simulink model "schemat_koncowy_irp"  (R2015a)
settings: Solver=ode1  StartTime=0.0  StopTime=Inf  FixedStep=0.001  RelTol=1e-3
PostLoadFcn:
  | , if any(exist('dsrtsu_mdlpostloadfcn', 'file') == [2, 3, 6]), try dsrtsu_mdlpostloadfcn('Execute', bdroot); catch fprintf('Error in PostLoadFcn (dsrtsu_mdlpostloadfcn) for model "%s":\n %s\n', bdroot, lasterr); end, end,
libraries: rtilibm x3
(part 1 of 2)
settings Model: DSRTSU_INTERNAL_RTI_VER=460  DSRTSU_INTERNAL_RTI_TYPE=rti1005  DSRTSU_INTERNAL_RTIFPGA=50  CovHtmlReporting=off  Creator=k21p930a  LastModifiedBy=k21p930a
settings OptimizationCC: BlockReduction=off  OptimizeBlockIOStorage=off  BufferReuse=off  GlobalBufferReuse=off  ExpressionFolding=off  LocalBlockOutputs=off
settings HardwareCC: ProdIntDivRoundTo=Zero  ProdEndianess=BigEndian  ProdHWDeviceType=Generic->Custom  TargetIntDivRoundTo=Zero  TargetEndianess=BigEndian  TargetHWDeviceType=Generic->Custom
settings RTWCC: SystemTargetFile=rti1005.tlc  MakeCommand=make_rti  TemplateMakefile=rti1005.tmf  Description=dSPACE DS1005 Hardware Platform
settings STFCustomTargetCC: GenerateSampleERTMain=off  ParMdlRefBuildCompliant=on  GeneratePreprocessorConditionals=Disable all  ERTCustomFileBanners=off  SupportNonInlinedSFcns=on  SupportVariableSizeSignals=off  MATLABClassNameForMDSCustomization=Simulink.SoftwareTarget.GRTCustomization  GRTInterface=on  SystemTargetFile=rti1005.tlc
settings GRTTargetCC: CompOptLevelCompliant=off  ConcurrentExecutionCompliant=off  CombineOutputUpdateFcns=off  MatFileLogging=off  CPPClassGenCompliant=off  GRTInterface=on  ExtModeMexFile=noextcomm

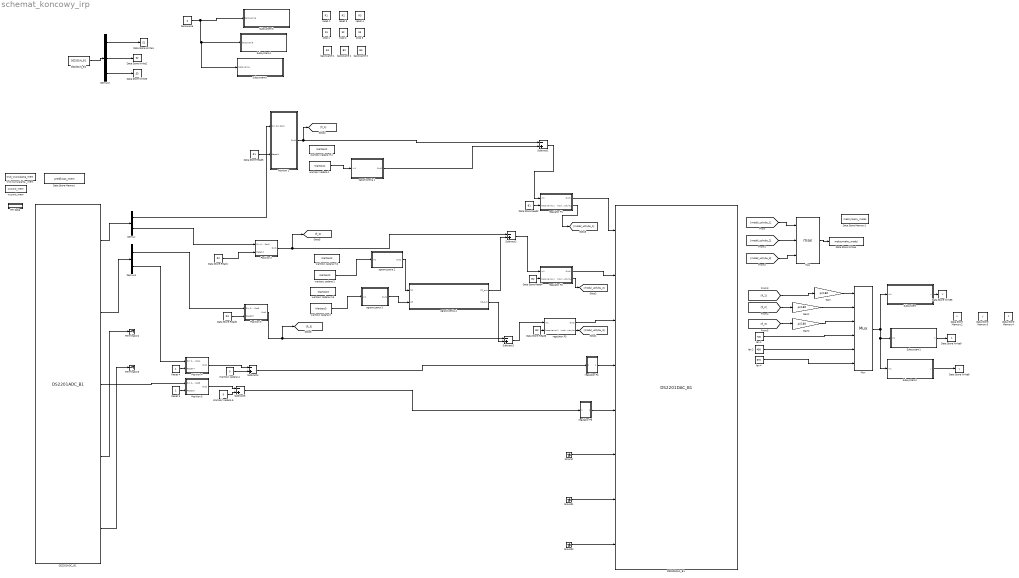
== system schemat_koncowy_irp ==
  DS2201ADC_B1 : rtilibm/DS2201/DS2201ADC_B1  BoardNo=1  channelNo1=[1 2 3 4]  channelNo2=[5 6 7 8]  channelNo3=[9 10]  channelNo4=-1  channelNo5=-1  DialogFcn=gui2201adc  UnitName={'DS2201ADC_B'}  UnitValues={ 1 }  DSProperties=struct('RTI',struct('Version',uint32(1),'BlockType',struct('isSLSource',uint8(1),'isSLSink',uint8(0),'isHWSource',uint8(1),'isHWSink',uint8(0),'isSetup',uint8(0),'isInline',uint8(1),'isNonInline',uint8(0),'isInterrupt',uint8(0),'isChannelwise',uint8(0)),'IOBoardType','DS2201','UnitType','ADC','Identifier','ADCMUX','DialogType','ML','BlockSet','NONE','SlaveProcessor','NONE'))
  DS2201DAC_B1 : rtilibm/DS2201/DS2201DAC_B1  BoardNo=1  IOErrorMode=[0 0]  InitValue=[0 0 0 0 0 0 0 0]  TermMode=[0 0 0 0 0 0 0 0]  TermValue=[0 0 0 0 0 0 0 0]  DialogFcn=gui2201dac  UnitName={'DS2201DAC_B'}  UnitValues={ 1 }  DSProperties=struct('RTI',struct('Version',uint32(1),'BlockType',struct('isSLSource',uint8(0),'isSLSink',uint8(1),'isHWSource',uint8(0),'isHWSink',uint8(1),'isSetup',uint8(0),'isInline',uint8(1),'isNonInline',uint8(0),'isInterrupt',uint8(0),'isChannelwise',uint8(0)),'IOBoardType','DS2201','UnitType','DAC','Identifier','DAC','DialogType','ML','BlockSet','NONE','SlaveProcessor','NONE'))
  DS2201IN_B1 : rtilibm/DS2201/DS2201IN_B1  BoardNo=1  ChannelNos=[1 2 3]  DialogFcn=gui2201in  UnitName={ 'DS2201IN_B' }  UnitValues={ 1 }  DSProperties=struct('RTI',struct('Version',uint32(1),'BlockType',struct('isSLSource',uint8(1),'isSLSink',uint8(0),'isHWSource',uint8(1),'isHWSink',uint8(0),'isSetup',uint8(0),'isInline',uint8(1),'isNonInline',uint8(0),'isInterrupt',uint8(0),'isChannelwise',uint8(0)),'IOBoardType','DS2201','UnitType','BIT','Identifier','BITIN','DialogType','ML','BlockSet','NONE','SlaveProcessor','NONE'))
  Data Store Memory : DataStoreMemory  DataStoreName=predkosc_mem  ReadBeforeWriteMsg=warning  WriteAfterWriteMsg=warning  WriteAfterReadMsg=warning  InitialValue=0.3
  Data Store Memory1 : DataStoreMemory  DataStoreName=maksymalny_modul  ReadBeforeWriteMsg=warning  WriteAfterWriteMsg=warning  WriteAfterReadMsg=warning
  Data Store Memory2 : DataStoreMemory  DataStoreName=x  ReadBeforeWriteMsg=warning  WriteAfterWriteMsg=warning  WriteAfterReadMsg=warning
  Data Store Memory3 : DataStoreMemory  DataStoreName=y  ReadBeforeWriteMsg=warning  WriteAfterWriteMsg=warning  WriteAfterReadMsg=warning
  Data Store Memory4 : DataStoreMemory  DataStoreName=z  ReadBeforeWriteMsg=warning  WriteAfterWriteMsg=warning  WriteAfterReadMsg=warning
  Data Store Read1 : DataStoreRead  DataStoreName=R2
  Data Store Read2 : DataStoreRead  DataStoreName=B1
  Data Store Read3 : DataStoreRead  DataStoreName=R3
  Data Store Read4 : DataStoreRead  DataStoreName=B2
  Data Store Read5 : DataStoreRead  DataStoreName=R1
  Data Store Read6 : DataStoreRead  DataStoreName=B3
  Data Store Write1 : DataStoreWrite  DataStoreName=S1
  Data Store Write2 : DataStoreWrite  DataStoreName=S2
  Data Store Write3 : DataStoreWrite  DataStoreName=S3
  Data Store Write4 : DataStoreWrite  DataStoreName=maksymalny_modul
  Data Store Write5 : DataStoreWrite  DataStoreName=x
  Data Store Write8 : DataStoreWrite  DataStoreName=y
  Data Store Write9 : DataStoreWrite  DataStoreName=z
  Demux : Demux  Outputs=2
  Demux1 : Demux  Outputs=2
  Demux2 : Demux  Outputs=3
  Gain : Gain  Gain=pi/180
  Gain1 : Gain  Gain=pi/180
  Gain2 : Gain  Gain=pi/180
  Ground : Ground
  Ground1 : Ground
  Ground2 : Ground
  Max : MinMax  Function=max  Inputs=3
  Mux : Mux  Inputs=6
  Position 1 : Subsystem
  Position 2 : Subsystem
  Position 3 : Subsystem
  Position 4 : Subsystem
  Position 5 : Subsystem
  RTI Data : Subsystem  Tag=struct('RTIDataServer',struct('RTIDataServerVs','2','RTIModelDescription','struct(''main'',''schemat_koncowy_irp'',''sub'',''schemat_koncowy_irp'',''isMp'',0)'))  LoadFcn="if exist('rtidc'), try,  rtidc('DataHostBlockClbLoad', gcbh); catch, disp(['Warning: ''LoadFcn'' for RTI Data block failed: ' lasterr]); end, end,"  mask(RTI_DATA_HOST){}
      mask help:
      | RTI Data Block.
      | This block is used by RTI to store internal model-dependent data.
      | Please keep this block on the root level of the model. Deleting this block will result in data loss.
      |
      | NEVER DELETE OR COPY THIS BLOCK!
      settings: CopyFcn="if exist('rtidc'), try,  rtidc('DataHostBlockClbCopy', gcbh); catch, disp(['Warning: ''CopyFcn'' for RTI Data block failed: ' lasterr]); end, end,"  DeleteFcn="if exist('rtidc'), try,  rtidc('DataHostBlockClbDelete', gcbh); catch, disp(['Warning: ''DeleteFcn'' for RTI Data block failed: ' lasterr]); end, end,"  ModelCloseFcn="if exist('rtidc'), try,  rtidc('DataHostBlockClbModelClose', gcbh); catch, disp(['Warning: ''ModelCloseFcn'' for RTI Data block failed: ' lasterr]); end, end,"  PreSaveFcn="if exist('rtidc'), try,  rtidc('DataHostBlockClbPreSave', gcbh); catch, disp(['Warning: ''PreSaveFcn'' for RTI Data block failed: ' lasterr]); end, end,"  PostSaveFcn="if exist('rtidc'), try,  rtidc('DataHostBlockClbPostSave', gcbh); catch, disp(['Warning: ''PostSaveFcn'' for RTI Data block failed: ' lasterr]); end, end,"  NameChangeFcn="if exist('rtidc'), try,  rtidc('DataHostBlockClbNameChange', gcbh); catch, disp(['Warning: ''NameChangeFcn'' for RTI Data block failed: ' lasterr]); end, end,"
      mask Help:
      | RTI Data Block.
      | This block is used by RTI to store internal model-dependent data.
      | Please keep this block on the root level of the model. Deleting this block will result in data loss.
      | 
      | NEVER DELETE OR COPY THIS BLOCK!
      mask Display:
      | text(0.5, 0.5, 'RTI Data', 'HorizontalAlignment', 'center');
      | plot([1 0]);
  Reset 4 : Constant
  Reset 5 : Constant
  Subsystem : Subsystem
  Subsystem1 : Subsystem
  Subsystem2 : Subsystem
  Subsystem3 : Subsystem
  Subsystem4 : Subsystem
  Subsystem5 : Subsystem
  Subtract{1..5} (5 alike) : Sum  Inputs=-+
  Terminator2 : Terminator
  Terminator3 : Terminator
  Wartość zadana 4 : Constant  Value=0
  Wartość zadana 5 : Constant  Value=0
  "bazowanie " : Constant  Value=0
  bazowanie 1 : DataStoreMemory  DataStoreName=B1  ReadBeforeWriteMsg=warning  WriteAfterWriteMsg=warning  WriteAfterReadMsg=warning
  bazowanie 2 : DataStoreMemory  DataStoreName=B2  ReadBeforeWriteMsg=warning  WriteAfterWriteMsg=warning  WriteAfterReadMsg=warning
  bazowanie 3 : DataStoreMemory  DataStoreName=B3  ReadBeforeWriteMsg=warning  WriteAfterWriteMsg=warning  WriteAfterReadMsg=warning
  len 1 : Constant  Value=700
  len 2 : Constant  Value=450
  len 4 : Constant  Value=670
  ograniczenia 1 : Subsystem
  ograniczenia 2 : Subsystem
  ograniczenia 3 : Subsystem
  ograniczenia 4 : Subsystem
  regulator P1 : Subsystem
  regulator P2 : Subsystem
  regulator P3 : Subsystem
  regulator P4 : Subsystem
  regulator P5 : Subsystem
  reset 1 : DataStoreMemory  DataStoreName=R1  ReadBeforeWriteMsg=warning  WriteAfterWriteMsg=warning  WriteAfterReadMsg=warning  OutDataTypeStr=double
  reset 3 : DataStoreMemory  DataStoreName=R2  ReadBeforeWriteMsg=warning  WriteAfterWriteMsg=warning  WriteAfterReadMsg=warning  OutDataTypeStr=double
  reset 4 : DataStoreMemory  DataStoreName=R3  ReadBeforeWriteMsg=warning  WriteAfterWriteMsg=warning  WriteAfterReadMsg=warning  OutDataTypeStr=double
  stop 1 : DataStoreMemory  DataStoreName=S1  ReadBeforeWriteMsg=warning  WriteAfterWriteMsg=warning  WriteAfterReadMsg=warning
  stop 2 : DataStoreMemory  DataStoreName=S2  ReadBeforeWriteMsg=warning  WriteAfterWriteMsg=warning  WriteAfterReadMsg=warning
  stop 3 : DataStoreMemory  DataStoreName=S3  ReadBeforeWriteMsg=warning  WriteAfterWriteMsg=warning  WriteAfterReadMsg=warning
  "tryb wyzwalania _mem " : DataStoreMemory  DataStoreName=tryb_wyzwalania_mem  ReadBeforeWriteMsg=warning  WriteAfterWriteMsg=warning  WriteAfterReadMsg=warning
  wartosc zadana 1 : DataStoreRead  DataStoreName=Wartosc1
  wartosc zadana 2 : DataStoreRead  DataStoreName=Wartosc2
  wartosc zadana 3 : DataStoreRead  DataStoreName=Wartosc3
  wartosc zadana m1 : DataStoreMemory  DataStoreName=Wartosc1  ReadBeforeWriteMsg=warning  WriteAfterWriteMsg=warning  WriteAfterReadMsg=warning
  wartosc zadana m2 : DataStoreMemory  DataStoreName=Wartosc2  ReadBeforeWriteMsg=warning  WriteAfterWriteMsg=warning  WriteAfterReadMsg=warning
  wartosc zadana m3 : DataStoreMemory  DataStoreName=Wartosc3  ReadBeforeWriteMsg=warning  WriteAfterWriteMsg=warning  WriteAfterReadMsg=warning
  wyzwol_mem : DataStoreMemory  DataStoreName=wyzwol_mem  ReadBeforeWriteMsg=warning  WriteAfterWriteMsg=warning  WriteAfterReadMsg=warning
  wires:
  Demux1/2 -> Position 4/1(Sin && Cos4)
  DS2201ADC_B1/1 -> Demux/1
  DS2201ADC_B1/2 -> Demux1/1
  DS2201ADC_B1/5 -> Terminator3/1
  DS2201ADC_B1/4 -> Terminator2/1
  Demux/1 -> Position 1/1(Sin && Cos1)
  Demux/2 -> Position 2/1(Sin && Cos2)
  Demux1/1 -> Position 3/1(Sin && Cos3)
  DS2201ADC_B1/3 -> Position 5/1(Sin && Cos5)
  regulator P1/1(Out1) -> DS2201DAC_B1/1
  regulator P4/1(Out1) -> DS2201DAC_B1/4
  regulator P5/1(Out1) -> DS2201DAC_B1/5
  wartosc zadana 1/1 -> ograniczenia 1/1(In1)
  Position 1/1(Out1) -> [fi_1], Subtract1/1
  Position 2/1(Out1) -> [fi_2], Subtract2/1
  Position 3/1(Out1) -> [fi_3], Subtract3/1
  Position 4/1(Out1) -> Subtract4/1
  Position 5/1(Out1) -> Subtract5/1
  Subtract5/1 -> regulator P5/1(In1)
  Subtract4/1 -> regulator P4/1(In1)
  Ground/1 -> DS2201DAC_B1/6
  Ground1/1 -> DS2201DAC_B1/7
  Ground2/1 -> DS2201DAC_B1/8
  Wartość zadana 4/1 -> Subtract4/2
  Wartość zadana 5/1 -> Subtract5/2
  Reset 4/1 -> Position 4/2(Reset 4)
  Reset 5/1 -> Position 5/2(Reset 5)
  DS2201IN_B1/1 -> Demux2/1
  ograniczenia 1/1(Out1) -> Subtract1/2
  Subtract1/1 -> regulator P1/1(In1)
  ograniczenia 2/1(Out1) -> ograniczenia 4/1(Z2)
  ograniczenia 4/1(Z2_out) -> Subtract2/2
  ograniczenia 3/1(Out1) -> ograniczenia 4/2(Z3)
  ograniczenia 4/2("Z3_out ") -> Subtract3/2
  Demux2/1 -> Data Store Write1/1
  Demux2/2 -> Data Store Write2/1
  Demux2/3 -> Data Store Write3/1
  Data Store Read3/1 -> Position 3/2(Reset 3)
  Data Store Read5/1 -> Position 1/2(Reset 1)
  Data Store Read2/1 -> regulator P1/2(bazowanie 1)
  regulator P2/1(Out1) -> DS2201DAC_B1/2
  Subtract2/1 -> regulator P2/1(In1)
  regulator P3/1(Out1) -> DS2201DAC_B1/3
  Subtract3/1 -> regulator P3/1(In1)
  regulator P3/2(modul uchybu) -> [modul_uchybu_3]
  regulator P2/2(modul uchybu) -> [modul_uchybu_2]
  regulator P1/2(modul uchybu) -> [modul_uchybu_1]
  [modul_uchybu_1] -> Max/1
  [modul_uchybu_2] -> Max/2
  [modul_uchybu_3] -> Max/3
  Max/1 -> Data Store Write4/1
  [fi_1] -> Gain/1
  [fi_2] -> Gain1/1
  [fi_3] -> Gain2/1
  len 1/1 -> Mux/4
  len 2/1 -> Mux/5
  len 4/1 -> Mux/6
  Mux/1 -> Subsystem/1(In1), Subsystem2/1(In1), Subsystem1/1(In1)
  Subsystem/1(x) -> Data Store Write5/1
  Subsystem2/1(y) -> Data Store Write8/1
  Gain1/1 -> Mux/2
  Gain2/1 -> Mux/3
  Gain/1 -> Mux/1
  "bazowanie "/1 -> Subsystem5/1(bazowanie), Subsystem4/1(bazowanie), Subsystem3/1(bazowanie)
  Data Store Read1/1 -> Position 2/2(Reset 2)
  Data Store Read4/1 -> regulator P2/2(bazowanie 1)
  Data Store Read6/1 -> regulator P3/2(bazowanie 1)
  wartosc zadana 3/1 -> ograniczenia 3/1(In1)
  wartosc zadana 2/1 -> ograniczenia 2/1(In1)
  Subsystem1/1(z) -> Data Store Write9/1

== system schemat_koncowy_irp/Position 1 ==
  Sin && Cos1 : Inport
  Reset 1 : Inport  Port=2
  Filters 1 : Subsystem
  Position Calculation 1 : Subsystem
  Out1 : Outport
  wires:
  Filters 1/1(Sin) -> Position Calculation 1/1(Sin)
  Filters 1/2(Cos) -> Position Calculation 1/2(Cos)
  Sin && Cos1/1 -> Filters 1/1(Sin && Cos)
  Reset 1/1 -> Position Calculation 1/3(Reset (Impulse))
  Position Calculation 1/1(Position) -> Out1/1

== system schemat_koncowy_irp/Position 2 ==
  Sin && Cos2 : Inport
  Reset 2 : Inport  Port=2
  Filters 2 : Subsystem
  Position Calculation 2 : Subsystem
  Out1 : Outport
  wires:
  Filters 2/1(Sin) -> Position Calculation 2/1(Sin)
  Filters 2/2(Cos) -> Position Calculation 2/2(Cos)
  Sin && Cos2/1 -> Filters 2/1(Sin && Cos)
  Reset 2/1 -> Position Calculation 2/3(Reset (Impulse))
  Position Calculation 2/1(Position) -> Out1/1

== system schemat_koncowy_irp/Position 3 ==
  Sin && Cos3 : Inport
  Reset 3 : Inport  Port=2
  Filters 3 : Subsystem
  Position Calculation 3 : Subsystem
  Out1 : Outport
  wires:
  Filters 3/1(Sin) -> Position Calculation 3/1(Sin)
  Filters 3/2(Cos) -> Position Calculation 3/2(Cos)
  Sin && Cos3/1 -> Filters 3/1(Sin && Cos)
  Reset 3/1 -> Position Calculation 3/3(Reset (Impulse))
  Position Calculation 3/1(Position) -> Out1/1

== system schemat_koncowy_irp/Position 4 ==
  Sin && Cos4 : Inport
  Reset 4 : Inport  Port=2
  Filters 4 : Subsystem
  Position Calculation 4 : Subsystem
  Out1 : Outport
  wires:
  Position Calculation 4/1(Position) -> Out1/1
  Reset 4/1 -> Position Calculation 4/3(Reset (Impulse))
  Sin && Cos4/1 -> Filters 4/1(Sin && Cos)
  Filters 4/2(Cos) -> Position Calculation 4/2(Cos)
  Filters 4/1(Sin) -> Position Calculation 4/1(Sin)

== system schemat_koncowy_irp/Position 5 ==
  Sin && Cos5 : Inport
  Reset 5 : Inport  Port=2
  Filters 5 : Subsystem
  Position Calculation 5 : Subsystem
  Out1 : Outport
  wires:
  Position Calculation 5/1(Position) -> Out1/1
  Reset 5/1 -> Position Calculation 5/3(Reset (Impulse))
  Sin && Cos5/1 -> Filters 5/1(Sin && Cos)
  Filters 5/2(Cos) -> Position Calculation 5/2(Cos)
  Filters 5/1(Sin) -> Position Calculation 5/1(Sin)

== system schemat_koncowy_irp/RTI Data ==
  RTI Data Store : Subsystem  Tag="struct('private',struct('version',struct('dsVer',uint32(2),'dsVerCreation',uint32(2),'RTI',struct('ver','7.4','type','RTI1005')),'access',struct('type','Model','isPerm',1,'created',['18-Oct-2021 10:10:05'],'modified',['08-Nov-2021 10:46:14'],'location','')),'public',struct('main',struct('data',[]),'sub',struct('name',{{'schemat_koncowy_irp'}},'data',{{struct('TH',struct('thTaskInfo',struct('taskType',{'TIMER','HWINT','TMRINT','SWINT','GLINT'},'tasksNumOf',{1,0,0,0,0},'srcIds',{{'TIMERA'},{},{},{},{}},'taskNames',{{['Timer Task 1']},{},{},{},{}})),'th_tc',struct('dataType','TASK','taskGroupId','','taskGroupList',{{}},'taskSchedulingPolicy','FCFS','taskType','TIMER','blkh',-1,'srcId','TIMERA','srcSgnName',['Timer A interrupt'],'srcCpuName','','taskName',['Timer Task 1  [0.001] s'],'taskNameDisplayExt','','smplTime',0.001,'smplTimeOffs',0,'hasFixedPriority',0,'priority',1,'hasFixedOvc',0,'ovcType',1,'ovcMax',1),'tc_th',struct('dataType','TASK','taskGroupId','','taskGroupList',{{}},'taskSchedulingPolicy','FCFS','taskType','TIMER','blkh',-1,'srcId','TIMERA','srcSgnName',['Timer A interrupt'],'srcCpuName','','taskName',['Timer Task 1  [0.001] s'],'taskNameDisplayExt','','smplTime',0.001,'smplTimeOffs',0,'hasFixedPriority',0,'priority',1,'hasFixedOvc',0,'ovcType',1,'ovcMax',1))}})))"  mask(RTI_DATA_STORE){}
      mask help:
      | RTI Data Store Block. This block is used by RTI to store internal model dependent data. Deleting this block will result in data loss.
      |
      | NEVER DELETE, COPY, OR MODIFY THIS BLOCK!
      mask Help:
      | RTI Data Store Block. This block is used by RTI to store internal model dependent data. Deleting this block will result in data loss.
      | 
      | NEVER DELETE, COPY, OR MODIFY THIS BLOCK!
      mask Display: text(0.5, 0.5, ' ', 'HorizontalAlignment', 'center');

== system schemat_koncowy_irp/Subsystem ==
  In1 : Inport
  Cos : Trigonometry  Operator=cos
  Cos1 : Trigonometry  Operator=cos
  Demux : Demux  Outputs=6
  Product : Product
  Product1 : Product
  Product2 : Product
  Sin : Trigonometry
  Sum : Sum  Inputs=|+-
  Sum1 : Sum  Inputs=|++
  Terminator : Terminator
  x : Outport
  wires:
  Cos/1 -> Product/1
  Sum/1 -> Product/2
  Product/1 -> x/1
  Demux/2 -> Sin/1, Sum1/1  "fi2-l"
  Demux/3 -> Sum1/2
  Sum1/1 -> Cos1/1
  Cos1/1 -> Product1/1
  Demux/6 -> Product1/2  "c"
  Product1/1 -> Sum/1
  Sin/1 -> Product2/1
  Demux/5 -> Product2/2  "b"
  Product2/1 -> Sum/2
  In1/1 -> Demux/1
  Demux/1 -> Cos/1  "fi1-k"
  Demux/4 -> Terminator/1

== system schemat_koncowy_irp/Subsystem1 ==
  In1 : Inport
  Cos : Trigonometry  Operator=cos
  Demux : Demux  Outputs=6
  Product : Product
  Product1 : Product
  Sin : Trigonometry
  Sum : Sum  Inputs=3
  Sum1 : Sum  Inputs=|++
  Terminator : Terminator
  z : Outport
  wires:
  Sum/1 -> z/1
  Demux/2 -> Sum1/1, Cos/1  "fi2-l"
  Demux/3 -> Sum1/2
  In1/1 -> Demux/1
  Demux/4 -> Sum/1
  Cos/1 -> Product/1
  Demux/5 -> Product/2  "b"
  Product/1 -> Sum/2
  Sum1/1 -> Sin/1
  Sin/1 -> Product1/1
  Demux/6 -> Product1/2  "c"
  Product1/1 -> Sum/3
  Demux/1 -> Terminator/1  "fi1-k"

== system schemat_koncowy_irp/Subsystem2 ==
  In1 : Inport
  Cos : Trigonometry  Operator=cos
  Demux : Demux  Outputs=6
  Minus : Sum  Inputs=+-
  Product : Product
  Product1 : Product
  Product2 : Product
  Sin : Trigonometry
  Sin1 : Trigonometry
  Sum : Sum  Inputs=|++
  Terminator : Terminator
  y : Outport
  wires:
  Demux/2 -> Sin1/1, Sum/1  "fi2-l"
  Demux/3 -> Sum/2
  In1/1 -> Demux/1
  Demux/1 -> Sin/1  "fi1-k"
  Demux/4 -> Terminator/1
  Sin/1 -> Product/1
  Minus/1 -> Product/2
  Sin1/1 -> Product1/1
  Demux/5 -> Product1/2  "b"
  Product1/1 -> Minus/1
  Sum/1 -> Cos/1
  Cos/1 -> Product2/1
  Demux/6 -> Product2/2  "c"
  Product2/1 -> Minus/2
  Product/1 -> y/1

== system schemat_koncowy_irp/Subsystem3 ==
  bazowanie : Inport
  01 : Constant  Value=0
  4 : Constant  Value=0
  Data Store Read : DataStoreRead  DataStoreName=B1
  Data Store Read1 : DataStoreRead  DataStoreName=B1
  Data Store Read2 : DataStoreRead  DataStoreName=S1
  Data Store Write : DataStoreWrite  DataStoreName=B1
  Data Store Write2 : DataStoreWrite  DataStoreName=R1
  Data Store Write3 : DataStoreWrite  DataStoreName=Wartosc1
  Data Type Conversion : DataTypeConversion  OutDataTypeStr=double
  NOT1 : Logic  Operator=NOT  IconShape=distinctive  AllPortsSameDT=off  OutDataTypeStr=boolean
  Switch : Switch  Criteria=u2 > Threshold
  Switch1 : Switch  Criteria=u2 > Threshold
  Switch4 : Switch  Criteria=u2 > Threshold
  wartosc zadana 1 : DataStoreRead  DataStoreName=Wartosc1
  wires:
  Switch1/1 -> Data Store Write/1
  4/1 -> Switch4/1
  bazowanie/1 -> Switch/2, Switch/1
  Data Store Read/1 -> Switch/3
  NOT1/1 -> Data Type Conversion/1
  Switch/1 -> Switch1/3
  01/1 -> Switch1/1
  Switch4/1 -> Data Store Write3/1
  wartosc zadana 1/1 -> Switch4/3
  Data Store Read1/1 -> Switch4/2, NOT1/1
  Data Store Read2/1 -> Switch1/2
  Data Type Conversion/1 -> Data Store Write2/1

== system schemat_koncowy_irp/Subsystem4 ==
  bazowanie : Inport
  01 : Constant  Value=0
  4 : Constant  Value=0
  Data Store Read : DataStoreRead  DataStoreName=B2
  Data Store Read1 : DataStoreRead  DataStoreName=B2
  Data Store Read2 : DataStoreRead  DataStoreName=S2
  Data Store Write : DataStoreWrite  DataStoreName=B2
  Data Store Write2 : DataStoreWrite  DataStoreName=R2
  Data Store Write3 : DataStoreWrite  DataStoreName=Wartosc2
  Data Type Conversion : DataTypeConversion  OutDataTypeStr=double
  NOT1 : Logic  Operator=NOT  IconShape=distinctive  AllPortsSameDT=off  OutDataTypeStr=boolean
  Switch : Switch  Criteria=u2 > Threshold
  Switch1 : Switch  Criteria=u2 > Threshold
  Switch4 : Switch  Criteria=u2 > Threshold
  wartosc zadana 2 : DataStoreRead  DataStoreName=Wartosc2
  wires:
  Switch1/1 -> Data Store Write/1
  4/1 -> Switch4/1
  bazowanie/1 -> Switch/2, Switch/1
  Data Store Read/1 -> Switch/3
  NOT1/1 -> Data Type Conversion/1
  Switch/1 -> Switch1/3
  01/1 -> Switch1/1
  Switch4/1 -> Data Store Write3/1
  wartosc zadana 2/1 -> Switch4/3
  Data Store Read1/1 -> Switch4/2, NOT1/1
  Data Store Read2/1 -> Switch1/2
  Data Type Conversion/1 -> Data Store Write2/1

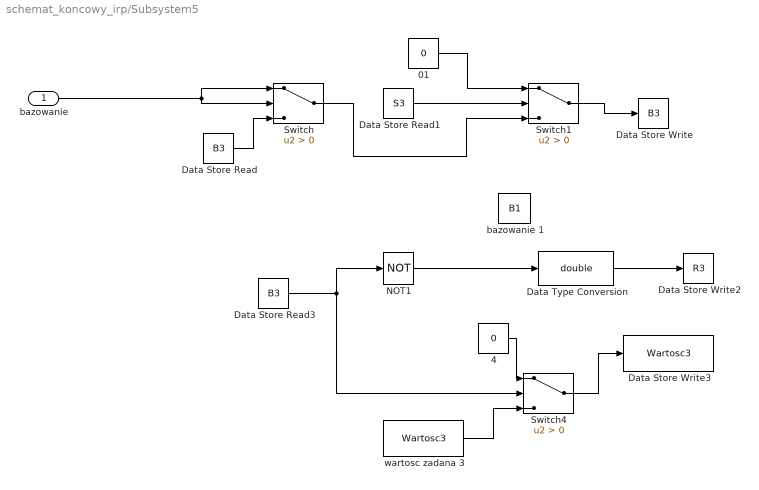
== system schemat_koncowy_irp/Subsystem5 ==
  bazowanie : Inport
  01 : Constant  Value=0
  4 : Constant  Value=0
  Data Store Read : DataStoreRead  DataStoreName=B3
  Data Store Read1 : DataStoreRead  DataStoreName=S3
  Data Store Read3 : DataStoreRead  DataStoreName=B3
  Data Store Write : DataStoreWrite  DataStoreName=B3
  Data Store Write2 : DataStoreWrite  DataStoreName=R3
  Data Store Write3 : DataStoreWrite  DataStoreName=Wartosc3
  Data Type Conversion : DataTypeConversion  OutDataTypeStr=double
  NOT1 : Logic  Operator=NOT  IconShape=distinctive  AllPortsSameDT=off  OutDataTypeStr=boolean
  Switch : Switch  Criteria=u2 > Threshold
  Switch1 : Switch  Criteria=u2 > Threshold
  Switch4 : Switch  Criteria=u2 > Threshold
  bazowanie 1 : DataStoreMemory  DataStoreName=B1  ReadBeforeWriteMsg=warning  WriteAfterWriteMsg=warning  WriteAfterReadMsg=warning
  wartosc zadana 3 : DataStoreRead  DataStoreName=Wartosc3
  wires:
  Switch1/1 -> Data Store Write/1
  4/1 -> Switch4/1
  bazowanie/1 -> Switch/2, Switch/1
  Data Store Read/1 -> Switch/3
  NOT1/1 -> Data Type Conversion/1
  Switch/1 -> Switch1/3
  01/1 -> Switch1/1
  Switch4/1 -> Data Store Write3/1
  wartosc zadana 3/1 -> Switch4/3
  Data Store Read3/1 -> NOT1/1, Switch4/2
  Data Store Read1/1 -> Switch1/2
  Data Type Conversion/1 -> Data Store Write2/1

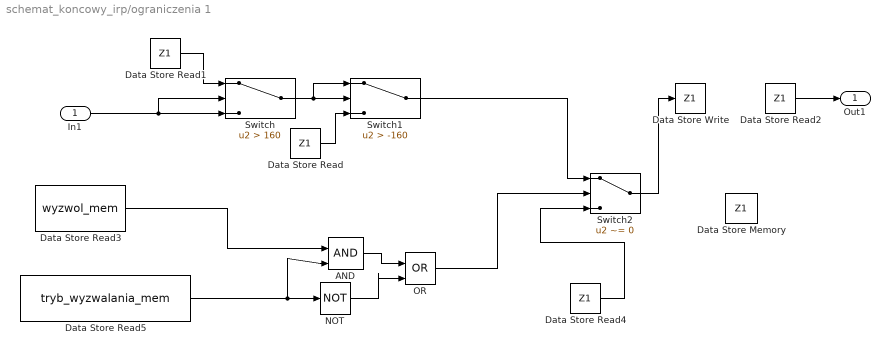
== system schemat_koncowy_irp/ograniczenia 1 ==
  In1 : Inport
  AND : Logic  IconShape=distinctive  AllPortsSameDT=off  OutDataTypeStr=boolean
  Data Store Memory : DataStoreMemory  DataStoreName=Z1  ReadBeforeWriteMsg=warning  WriteAfterWriteMsg=warning  WriteAfterReadMsg=warning
  Data Store Read{,1..2,4} (4 alike) : DataStoreRead  DataStoreName=Z1
  Data Store Read3 : DataStoreRead  DataStoreName=wyzwol_mem
  Data Store Read5 : DataStoreRead  DataStoreName=tryb_wyzwalania_mem
  Data Store Write : DataStoreWrite  DataStoreName=Z1
  NOT : Logic  Operator=NOT  IconShape=distinctive  AllPortsSameDT=off  OutDataTypeStr=boolean
  OR : Logic  Operator=OR  IconShape=distinctive  AllPortsSameDT=off  OutDataTypeStr=boolean
  Switch : Switch  Criteria=u2 > Threshold  Threshold=160
  Switch1 : Switch  Criteria=u2 > Threshold  Threshold=-160
  Switch2 : Switch  Criteria=u2 ~= 0  Threshold=-160
  Out1 : Outport
  wires:
  Switch/1 -> Switch1/1, Switch1/2
  In1/1 -> Switch/2, Switch/3
  Data Store Read/1 -> Switch1/3
  Data Store Read1/1 -> Switch/1
  Data Store Read2/1 -> Out1/1
  Data Store Read5/1 -> NOT/1, AND/2
  Switch2/1 -> Data Store Write/1
  Data Store Read3/1 -> AND/1
  AND/1 -> OR/1
  NOT/1 -> OR/2
  OR/1 -> Switch2/2
  Switch1/1 -> Switch2/1
  Data Store Read4/1 -> Switch2/3

== system schemat_koncowy_irp/ograniczenia 2 ==
  In1 : Inport
  AND : Logic  IconShape=distinctive  AllPortsSameDT=off  OutDataTypeStr=boolean
  Data Store Memory : DataStoreMemory  DataStoreName=Z2  ReadBeforeWriteMsg=warning  WriteAfterWriteMsg=warning  WriteAfterReadMsg=warning
  Data Store Read{,1..3} (4 alike) : DataStoreRead  DataStoreName=Z2
  Data Store Read4 : DataStoreRead  DataStoreName=wyzwol_mem
  Data Store Read5 : DataStoreRead  DataStoreName=tryb_wyzwalania_mem
  Data Store Write : DataStoreWrite  DataStoreName=Z2
  NOT : Logic  Operator=NOT  IconShape=distinctive  AllPortsSameDT=off  OutDataTypeStr=boolean
  OR : Logic  Operator=OR  IconShape=distinctive  AllPortsSameDT=off  OutDataTypeStr=boolean
  Switch : Switch  Criteria=u2 > Threshold  Threshold=40
  Switch1 : Switch  Criteria=u2 > Threshold  Threshold=-40
  Switch2 : Switch  Criteria=u2 ~= 0  Threshold=-160
  Out1 : Outport
  wires:
  Switch/1 -> Switch1/2, Switch1/1
  In1/1 -> Switch/2, Switch/3
  Data Store Read/1 -> Switch1/3
  Data Store Read1/1 -> Switch/1
  Data Store Read2/1 -> Out1/1
  NOT/1 -> OR/2
  Data Store Read3/1 -> Switch2/3
  AND/1 -> OR/1
  Switch2/1 -> Data Store Write/1
  Data Store Read5/1 -> NOT/1, AND/2
  OR/1 -> Switch2/2
  Data Store Read4/1 -> AND/1
  Switch1/1 -> Switch2/1

== system schemat_koncowy_irp/ograniczenia 3 ==
  In1 : Inport
  AND : Logic  IconShape=distinctive  AllPortsSameDT=off  OutDataTypeStr=boolean
  Data Store Memory : DataStoreMemory  DataStoreName=Z3  ReadBeforeWriteMsg=warning  WriteAfterWriteMsg=warning  WriteAfterReadMsg=warning
  Data Store Read{,1..3} (4 alike) : DataStoreRead  DataStoreName=Z3
  Data Store Read4 : DataStoreRead  DataStoreName=wyzwol_mem
  Data Store Read5 : DataStoreRead  DataStoreName=tryb_wyzwalania_mem
  Data Store Write : DataStoreWrite  DataStoreName=Z3
  NOT : Logic  Operator=NOT  IconShape=distinctive  AllPortsSameDT=off  OutDataTypeStr=boolean
  OR : Logic  Operator=OR  IconShape=distinctive  AllPortsSameDT=off  OutDataTypeStr=boolean
  Switch : Switch  Criteria=u2 > Threshold  Threshold=40
  Switch1 : Switch  Criteria=u2 > Threshold  Threshold=-25
  Switch2 : Switch  Criteria=u2 ~= 0  Threshold=-160
  Out1 : Outport
  wires:
  Switch/1 -> Switch1/2, Switch1/1
  In1/1 -> Switch/2, Switch/3
  Data Store Read/1 -> Switch1/3
  Data Store Read1/1 -> Switch/1
  Data Store Read2/1 -> Out1/1
  NOT/1 -> OR/2
  AND/1 -> OR/1
  Data Store Read3/1 -> Switch2/3
  Switch2/1 -> Data Store Write/1
  Data Store Read5/1 -> NOT/1, AND/2
  OR/1 -> Switch2/2
  Data Store Read4/1 -> AND/1
  Switch1/1 -> Switch2/1

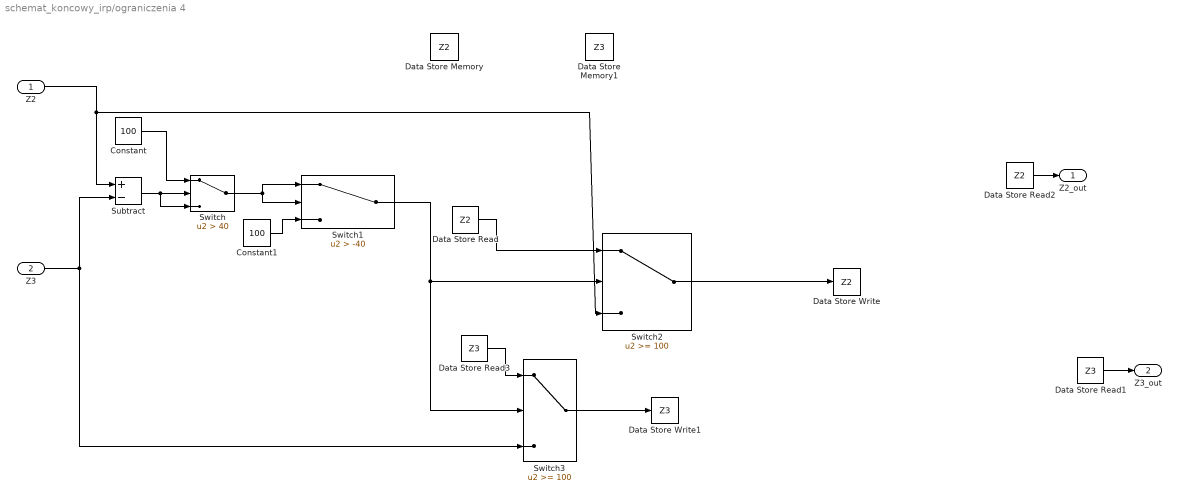
== system schemat_koncowy_irp/ograniczenia 4 ==
  Z2 : Inport
  Z3 : Inport  Port=2
  Constant : Constant  Value=100
  Constant1 : Constant  Value=100
  Data Store Memory : DataStoreMemory  DataStoreName=Z2  ReadBeforeWriteMsg=warning  WriteAfterWriteMsg=warning  WriteAfterReadMsg=warning
  Data Store Memory1 : DataStoreMemory  DataStoreName=Z3  ReadBeforeWriteMsg=warning  WriteAfterWriteMsg=warning  WriteAfterReadMsg=warning
  Data Store Read : DataStoreRead  DataStoreName=Z2
  Data Store Read1 : DataStoreRead  DataStoreName=Z3
  Data Store Read2 : DataStoreRead  DataStoreName=Z2
  Data Store Read3 : DataStoreRead  DataStoreName=Z3
  Data Store Write : DataStoreWrite  DataStoreName=Z2
  Data Store Write1 : DataStoreWrite  DataStoreName=Z3
  Subtract : Sum  Inputs=+-
  Switch : Switch  Criteria=u2 > Threshold  Threshold=40
  Switch1 : Switch  Criteria=u2 > Threshold  Threshold=-40
  Switch2 : Switch  Threshold=100
  Switch3 : Switch  Threshold=100
  Z2_out : Outport
  "Z3_out " : Outport  Port=2
  wires:
  Switch2/1 -> Data Store Write/1
  Z3/1 -> Subtract/2, Switch3/3
  Switch/1 -> Switch1/1, Switch1/2
  Subtract/1 -> Switch/3, Switch/2
  Data Store Read1/1 -> "Z3_out "/1
  Constant/1 -> Switch/1
  Constant1/1 -> Switch1/3
  Switch1/1 -> Switch3/2, Switch2/2
  Data Store Read/1 -> Switch2/1
  Data Store Read3/1 -> Switch3/1
  Z2/1 -> Subtract/1, Switch2/3
  Data Store Read2/1 -> Z2_out/1
  Switch3/1 -> Data Store Write1/1

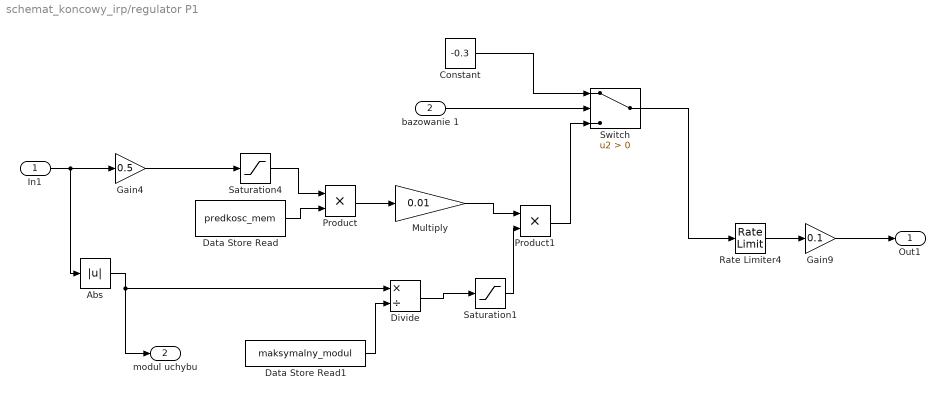
== system schemat_koncowy_irp/regulator P1 ==
  In1 : Inport
  bazowanie 1 : Inport  Port=2
  Abs : Abs
  Constant : Constant  Value=-0.3
  Data Store Read : DataStoreRead  DataStoreName=predkosc_mem
  Data Store Read1 : DataStoreRead  DataStoreName=maksymalny_modul
  Divide : Product  Inputs=*/
  Gain4 : Gain  Gain=0.5
  Gain9 : Gain  Gain=0.1
  Multiply : Gain  Gain=0.01
  Product : Product
  Product1 : Product
  Rate Limiter4 : RateLimiter  RisingSlewLimit=50  FallingSlewLimit=-50  SampleTimeMode=inherited
  Saturation1 : Saturate  UpperLimit=1  LowerLimit=0.001
  Saturation4 : Saturate  UpperLimit=3  LowerLimit=-3
  Switch : Switch  Criteria=u2 > Threshold
  Out1 : Outport
  modul uchybu : Outport  Port=2
  wires:
  In1/1 -> Abs/1, Gain4/1
  Gain4/1 -> Saturation4/1
  Rate Limiter4/1 -> Gain9/1
  Gain9/1 -> Out1/1
  bazowanie 1/1 -> Switch/2
  Constant/1 -> Switch/1
  Switch/1 -> Rate Limiter4/1
  Saturation4/1 -> Product/1
  Product/1 -> Multiply/1
  Data Store Read/1 -> Product/2
  Abs/1 -> Divide/1, modul uchybu/1
  Data Store Read1/1 -> Divide/2
  Divide/1 -> Saturation1/1
  Saturation1/1 -> Product1/2
  Multiply/1 -> Product1/1
  Product1/1 -> Switch/3

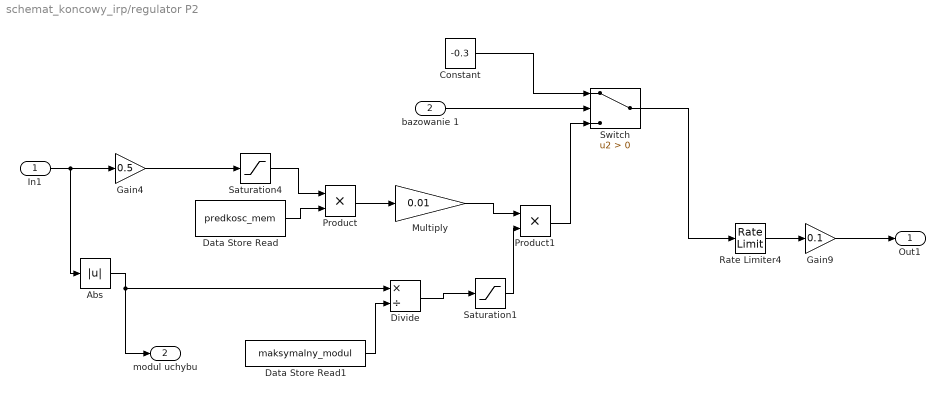
== system schemat_koncowy_irp/regulator P2 ==
  In1 : Inport
  bazowanie 1 : Inport  Port=2
  Abs : Abs
  Constant : Constant  Value=-0.3
  Data Store Read : DataStoreRead  DataStoreName=predkosc_mem
  Data Store Read1 : DataStoreRead  DataStoreName=maksymalny_modul
  Divide : Product  Inputs=*/
  Gain4 : Gain  Gain=0.5
  Gain9 : Gain  Gain=0.1
  Multiply : Gain  Gain=0.01
  Product : Product
  Product1 : Product
  Rate Limiter4 : RateLimiter  RisingSlewLimit=50  FallingSlewLimit=-50  SampleTimeMode=inherited
  Saturation1 : Saturate  UpperLimit=1  LowerLimit=0.001
  Saturation4 : Saturate  UpperLimit=3  LowerLimit=-3
  Switch : Switch  Criteria=u2 > Threshold
  Out1 : Outport
  modul uchybu : Outport  Port=2
  wires:
  In1/1 -> Abs/1, Gain4/1
  Gain4/1 -> Saturation4/1
  Rate Limiter4/1 -> Gain9/1
  Gain9/1 -> Out1/1
  bazowanie 1/1 -> Switch/2
  Constant/1 -> Switch/1
  Switch/1 -> Rate Limiter4/1
  Saturation4/1 -> Product/1
  Product/1 -> Multiply/1
  Data Store Read/1 -> Product/2
  Abs/1 -> Divide/1, modul uchybu/1
  Data Store Read1/1 -> Divide/2
  Divide/1 -> Saturation1/1
  Saturation1/1 -> Product1/2
  Multiply/1 -> Product1/1
  Product1/1 -> Switch/3

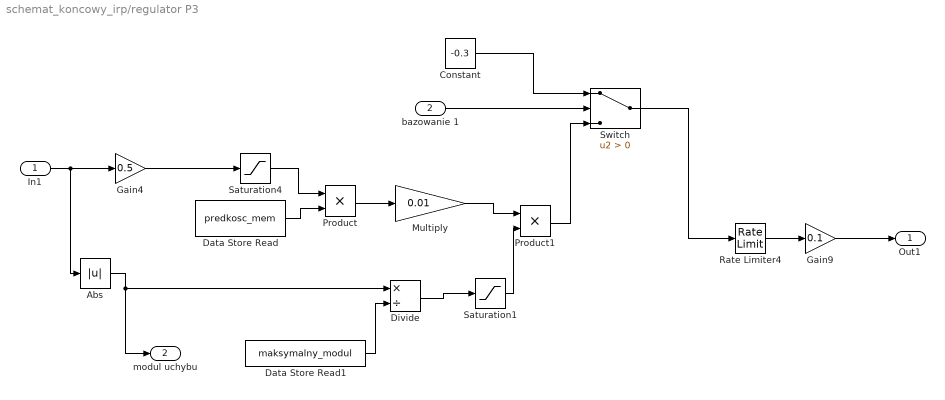
== system schemat_koncowy_irp/regulator P3 ==
  In1 : Inport
  bazowanie 1 : Inport  Port=2
  Abs : Abs
  Constant : Constant  Value=-0.3
  Data Store Read : DataStoreRead  DataStoreName=predkosc_mem
  Data Store Read1 : DataStoreRead  DataStoreName=maksymalny_modul
  Divide : Product  Inputs=*/
  Gain4 : Gain  Gain=0.5
  Gain9 : Gain  Gain=0.1
  Multiply : Gain  Gain=0.01
  Product : Product
  Product1 : Product
  Rate Limiter4 : RateLimiter  RisingSlewLimit=50  FallingSlewLimit=-50  SampleTimeMode=inherited
  Saturation1 : Saturate  UpperLimit=1  LowerLimit=0.001
  Saturation4 : Saturate  UpperLimit=3  LowerLimit=-3
  Switch : Switch  Criteria=u2 > Threshold
  Out1 : Outport
  modul uchybu : Outport  Port=2
  wires:
  In1/1 -> Abs/1, Gain4/1
  Gain4/1 -> Saturation4/1
  Rate Limiter4/1 -> Gain9/1
  Gain9/1 -> Out1/1
  bazowanie 1/1 -> Switch/2
  Constant/1 -> Switch/1
  Switch/1 -> Rate Limiter4/1
  Saturation4/1 -> Product/1
  Product/1 -> Multiply/1
  Data Store Read/1 -> Product/2
  Abs/1 -> Divide/1, modul uchybu/1
  Data Store Read1/1 -> Divide/2
  Divide/1 -> Saturation1/1
  Saturation1/1 -> Product1/2
  Multiply/1 -> Product1/1
  Product1/1 -> Switch/3

== system schemat_koncowy_irp/regulator P4 ==
  In1 : Inport
  Gain4 : Gain  Gain=0.5
  Gain9 : Gain  Gain=0.1
  Rate Limiter4 : RateLimiter  RisingSlewLimit=50  FallingSlewLimit=-50  SampleTimeMode=inherited
  Saturation4 : Saturate  UpperLimit=3  LowerLimit=-3
  Out1 : Outport
  wires:
  In1/1 -> Gain4/1
  Gain4/1 -> Saturation4/1
  Saturation4/1 -> Rate Limiter4/1
  Rate Limiter4/1 -> Gain9/1
  Gain9/1 -> Out1/1

== system schemat_koncowy_irp/regulator P5 ==
  In1 : Inport
  Gain4 : Gain  Gain=0.5
  Gain9 : Gain  Gain=0.1
  Rate Limiter4 : RateLimiter  RisingSlewLimit=50  FallingSlewLimit=-50  SampleTimeMode=inherited
  Saturation4 : Saturate  UpperLimit=3  LowerLimit=-3
  Out1 : Outport
  wires:
  In1/1 -> Gain4/1
  Gain4/1 -> Saturation4/1
  Saturation4/1 -> Rate Limiter4/1
  Rate Limiter4/1 -> Gain9/1
  Gain9/1 -> Out1/1

== system schemat_koncowy_irp/Position 1/Filters 1 ==
  Sin && Cos : Inport
  Analog Butterworth LP Filter : Subsystem  mask(buttap){Parameter3=2*pi*16, Parameter4=1}
      mask prompts: Parameter3 "Cutoff frequency (rad/sec)"; Parameter4 "Order"
      mask help:
      | Analog Butterworth low pass filter.
      |
      | (Requires Signal Processing Toolbox)
      mask init:
      | [z,p,k]=buttap(@2); z=@1*z; p=@1*p; k=real(prod(-p)); [num,den]=zp2tf(z,p,k); w=logspace(log10(@1/10),log10(10*@1),20); h=freqs(num,den,w);
      mask Help: Butterworth low pass filter using MATLAB's butter command.
      mask Display: plot(20*log10(w),20*log10(abs(h)))
  Analog Butterworth LP Filter1 : Subsystem  mask(buttap){Parameter3=2*pi*16, Parameter4=1}
      mask prompts: Parameter3 "Cutoff frequency (rad/sec)"; Parameter4 "Order"
      mask help:
      | Analog Butterworth low pass filter.
      |
      | (Requires Signal Processing Toolbox)
      mask init:
      | [z,p,k]=buttap(@2); z=@1*z; p=@1*p; k=real(prod(-p)); [num,den]=zp2tf(z,p,k); w=logspace(log10(@1/10),log10(10*@1),20); h=freqs(num,den,w);
      mask Help: Butterworth low pass filter using MATLAB's butter command.
      mask Display: plot(20*log10(w),20*log10(abs(h)))
  Demux : Demux  Outputs=2
  Sin : Outport
  Cos : Outport  Port=2
  wires:
  Demux/2 -> Analog Butterworth LP Filter1/1(In1)
  Demux/1 -> Analog Butterworth LP Filter/1(In1)
  Sin && Cos/1 -> Demux/1
  Analog Butterworth LP Filter1/1(Out1) -> Cos/1
  Analog Butterworth LP Filter/1(Out1) -> Sin/1

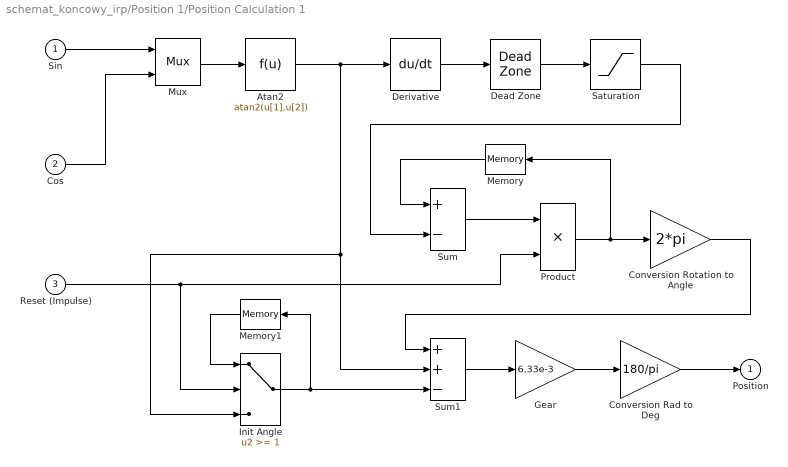
== system schemat_koncowy_irp/Position 1/Position Calculation 1 ==
  Sin : Inport
  Cos : Inport  Port=2
  Reset (Impulse) : Inport  Port=3
  Atan2 : Fcn  Expr=atan2(u[1],u[2])
  Conversion Rad to Deg : Gain  Gain=180/pi  SaturateOnIntegerOverflow=on  OutDataTypeStr=Inherit: Same as input  ParamDataTypeStr=Inherit: Same as input
  Conversion Rotation to Angle : Gain  Gain=2*pi  SaturateOnIntegerOverflow=on  OutDataTypeStr=Inherit: Same as input  ParamDataTypeStr=Inherit: Same as input
  Dead Zone : DeadZone  LowerValue=-5000  UpperValue=5000  SaturateOnIntegerOverflow=on
  Derivative : Derivative
  Gear : Gain  Gain=6.33e-3  SaturateOnIntegerOverflow=on  OutDataTypeStr=Inherit: Same as input  ParamDataTypeStr=Inherit: Same as input
  Init Angle : Switch  Threshold=1  SaturateOnIntegerOverflow=on  InputSameDT=on
  Memory : Memory
  Memory1 : Memory
  Mux : Mux  Inputs=2
  Product : Product  SaturateOnIntegerOverflow=on  RndMeth=Zero  InputSameDT=on  OutDataTypeStr=Inherit: Same as first input
  Saturation : Saturate  UpperLimit=1  LowerLimit=-1
  Sum : Sum  Inputs=+-  SaturateOnIntegerOverflow=on  InputSameDT=on  OutDataTypeStr=Inherit: Same as first input
  Sum1 : Sum  Inputs=++-  SaturateOnIntegerOverflow=on  InputSameDT=on  OutDataTypeStr=Inherit: Same as first input
  Position : Outport
  wires:
  Init Angle/1 -> Memory1/1, Sum1/3
  Memory1/1 -> Init Angle/1
  Product/1 -> Memory/1, Conversion Rotation to Angle/1
  Memory/1 -> Sum/1
  Cos/1 -> Mux/2
  Atan2/1 -> Init Angle/3, Sum1/2, Derivative/1
  Reset (Impulse)/1 -> Init Angle/2, Product/2
  Conversion Rotation to Angle/1 -> Sum1/1
  Saturation/1 -> Sum/2
  Conversion Rad to Deg/1 -> Position/1
  Sin/1 -> Mux/1
  Mux/1 -> Atan2/1
  Derivative/1 -> Dead Zone/1
  Dead Zone/1 -> Saturation/1
  Sum/1 -> Product/1
  Sum1/1 -> Gear/1
  Gear/1 -> Conversion Rad to Deg/1

== system schemat_koncowy_irp/Position 2/Filters 2 ==
  Sin && Cos : Inport
  Analog Butterworth LP Filter : Subsystem  mask(buttap){Parameter3=2*pi*16, Parameter4=1}
      mask prompts: Parameter3 "Cutoff frequency (rad/sec)"; Parameter4 "Order"
      mask help:
      | Analog Butterworth low pass filter.
      |
      | (Requires Signal Processing Toolbox)
      mask init:
      | [z,p,k]=buttap(@2); z=@1*z; p=@1*p; k=real(prod(-p)); [num,den]=zp2tf(z,p,k); w=logspace(log10(@1/10),log10(10*@1),20); h=freqs(num,den,w);
      mask Help: Butterworth low pass filter using MATLAB's butter command.
      mask Display: plot(20*log10(w),20*log10(abs(h)))
  Analog Butterworth LP Filter1 : Subsystem  mask(buttap){Parameter3=2*pi*16, Parameter4=1}
      mask prompts: Parameter3 "Cutoff frequency (rad/sec)"; Parameter4 "Order"
      mask help:
      | Analog Butterworth low pass filter.
      |
      | (Requires Signal Processing Toolbox)
      mask init:
      | [z,p,k]=buttap(@2); z=@1*z; p=@1*p; k=real(prod(-p)); [num,den]=zp2tf(z,p,k); w=logspace(log10(@1/10),log10(10*@1),20); h=freqs(num,den,w);
      mask Help: Butterworth low pass filter using MATLAB's butter command.
      mask Display: plot(20*log10(w),20*log10(abs(h)))
  Demux : Demux  Outputs=2
  Sin : Outport
  Cos : Outport  Port=2
  wires:
  Demux/2 -> Analog Butterworth LP Filter1/1(In1)
  Demux/1 -> Analog Butterworth LP Filter/1(In1)
  Sin && Cos/1 -> Demux/1
  Analog Butterworth LP Filter1/1(Out1) -> Cos/1
  Analog Butterworth LP Filter/1(Out1) -> Sin/1

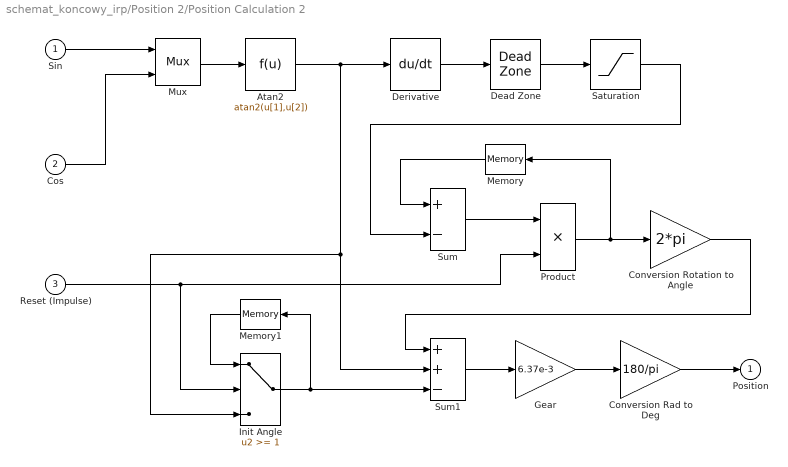
== system schemat_koncowy_irp/Position 2/Position Calculation 2 ==
  Sin : Inport
  Cos : Inport  Port=2
  Reset (Impulse) : Inport  Port=3
  Atan2 : Fcn  Expr=atan2(u[1],u[2])
  Conversion Rad to Deg : Gain  Gain=180/pi  SaturateOnIntegerOverflow=on  OutDataTypeStr=Inherit: Same as input  ParamDataTypeStr=Inherit: Same as input
  Conversion Rotation to Angle : Gain  Gain=2*pi  SaturateOnIntegerOverflow=on  OutDataTypeStr=Inherit: Same as input  ParamDataTypeStr=Inherit: Same as input
  Dead Zone : DeadZone  LowerValue=-5000  UpperValue=5000  SaturateOnIntegerOverflow=on
  Derivative : Derivative
  Gear : Gain  Gain=6.37e-3  SaturateOnIntegerOverflow=on  OutDataTypeStr=Inherit: Same as input  ParamDataTypeStr=Inherit: Same as input
  Init Angle : Switch  Threshold=1  SaturateOnIntegerOverflow=on  InputSameDT=on
  Memory : Memory
  Memory1 : Memory
  Mux : Mux  Inputs=2
  Product : Product  SaturateOnIntegerOverflow=on  RndMeth=Zero  InputSameDT=on  OutDataTypeStr=Inherit: Same as first input
  Saturation : Saturate  UpperLimit=1  LowerLimit=-1
  Sum : Sum  Inputs=+-  SaturateOnIntegerOverflow=on  InputSameDT=on  OutDataTypeStr=Inherit: Same as first input
  Sum1 : Sum  Inputs=++-  SaturateOnIntegerOverflow=on  InputSameDT=on  OutDataTypeStr=Inherit: Same as first input
  Position : Outport
  wires:
  Init Angle/1 -> Memory1/1, Sum1/3
  Memory1/1 -> Init Angle/1
  Product/1 -> Memory/1, Conversion Rotation to Angle/1
  Memory/1 -> Sum/1
  Cos/1 -> Mux/2
  Atan2/1 -> Init Angle/3, Sum1/2, Derivative/1
  Reset (Impulse)/1 -> Init Angle/2, Product/2
  Conversion Rotation to Angle/1 -> Sum1/1
  Saturation/1 -> Sum/2
  Conversion Rad to Deg/1 -> Position/1
  Sin/1 -> Mux/1
  Mux/1 -> Atan2/1
  Derivative/1 -> Dead Zone/1
  Dead Zone/1 -> Saturation/1
  Sum/1 -> Product/1
  Sum1/1 -> Gear/1
  Gear/1 -> Conversion Rad to Deg/1

== system schemat_koncowy_irp/Position 3/Filters 3 ==
  Sin && Cos : Inport
  Analog Butterworth LP Filter : Subsystem  mask(buttap){Parameter3=2*pi*16, Parameter4=1}
      mask prompts: Parameter3 "Cutoff frequency (rad/sec)"; Parameter4 "Order"
      mask help:
      | Analog Butterworth low pass filter.
      |
      | (Requires Signal Processing Toolbox)
      mask init:
      | [z,p,k]=buttap(@2); z=@1*z; p=@1*p; k=real(prod(-p)); [num,den]=zp2tf(z,p,k); w=logspace(log10(@1/10),log10(10*@1),20); h=freqs(num,den,w);
      mask Help: Butterworth low pass filter using MATLAB's butter command.
      mask Display: plot(20*log10(w),20*log10(abs(h)))
  Analog Butterworth LP Filter1 : Subsystem  mask(buttap){Parameter3=2*pi*16, Parameter4=1}
      mask prompts: Parameter3 "Cutoff frequency (rad/sec)"; Parameter4 "Order"
      mask help:
      | Analog Butterworth low pass filter.
      |
      | (Requires Signal Processing Toolbox)
      mask init:
      | [z,p,k]=buttap(@2); z=@1*z; p=@1*p; k=real(prod(-p)); [num,den]=zp2tf(z,p,k); w=logspace(log10(@1/10),log10(10*@1),20); h=freqs(num,den,w);
      mask Help: Butterworth low pass filter using MATLAB's butter command.
      mask Display: plot(20*log10(w),20*log10(abs(h)))
  Demux : Demux  Outputs=2
  Sin : Outport
  Cos : Outport  Port=2
  wires:
  Demux/2 -> Analog Butterworth LP Filter1/1(In1)
  Demux/1 -> Analog Butterworth LP Filter/1(In1)
  Sin && Cos/1 -> Demux/1
  Analog Butterworth LP Filter1/1(Out1) -> Cos/1
  Analog Butterworth LP Filter/1(Out1) -> Sin/1

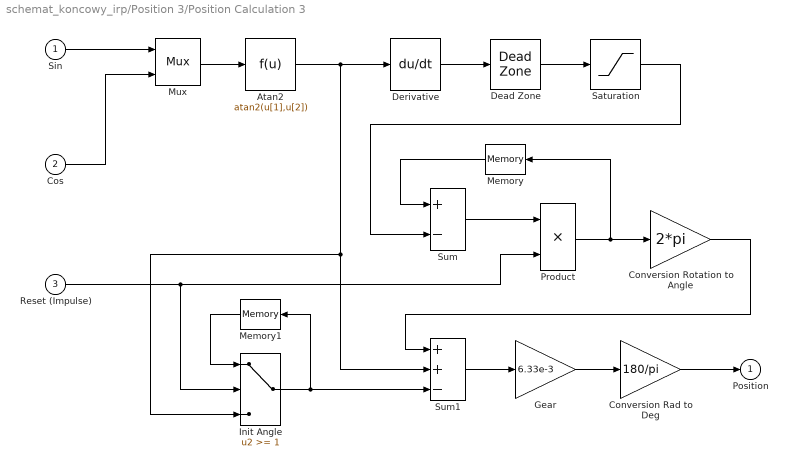
== system schemat_koncowy_irp/Position 3/Position Calculation 3 ==
  Sin : Inport
  Cos : Inport  Port=2
  Reset (Impulse) : Inport  Port=3
  Atan2 : Fcn  Expr=atan2(u[1],u[2])
  Conversion Rad to Deg : Gain  Gain=180/pi  SaturateOnIntegerOverflow=on  OutDataTypeStr=Inherit: Same as input  ParamDataTypeStr=Inherit: Same as input
  Conversion Rotation to Angle : Gain  Gain=2*pi  SaturateOnIntegerOverflow=on  OutDataTypeStr=Inherit: Same as input  ParamDataTypeStr=Inherit: Same as input
  Dead Zone : DeadZone  LowerValue=-5000  UpperValue=5000  SaturateOnIntegerOverflow=on
  Derivative : Derivative
  Gear : Gain  Gain=6.33e-3  SaturateOnIntegerOverflow=on  OutDataTypeStr=Inherit: Same as input  ParamDataTypeStr=Inherit: Same as input
  Init Angle : Switch  Threshold=1  SaturateOnIntegerOverflow=on  InputSameDT=on
  Memory : Memory
  Memory1 : Memory
  Mux : Mux  Inputs=2
  Product : Product  SaturateOnIntegerOverflow=on  RndMeth=Zero  InputSameDT=on  OutDataTypeStr=Inherit: Same as first input
  Saturation : Saturate  UpperLimit=1  LowerLimit=-1
  Sum : Sum  Inputs=+-  SaturateOnIntegerOverflow=on  InputSameDT=on  OutDataTypeStr=Inherit: Same as first input
  Sum1 : Sum  Inputs=++-  SaturateOnIntegerOverflow=on  InputSameDT=on  OutDataTypeStr=Inherit: Same as first input
  Position : Outport
  wires:
  Init Angle/1 -> Memory1/1, Sum1/3
  Memory1/1 -> Init Angle/1
  Product/1 -> Memory/1, Conversion Rotation to Angle/1
  Memory/1 -> Sum/1
  Cos/1 -> Mux/2
  Atan2/1 -> Init Angle/3, Sum1/2, Derivative/1
  Reset (Impulse)/1 -> Init Angle/2, Product/2
  Conversion Rotation to Angle/1 -> Sum1/1
  Saturation/1 -> Sum/2
  Conversion Rad to Deg/1 -> Position/1
  Sin/1 -> Mux/1
  Mux/1 -> Atan2/1
  Derivative/1 -> Dead Zone/1
  Dead Zone/1 -> Saturation/1
  Sum/1 -> Product/1
  Sum1/1 -> Gear/1
  Gear/1 -> Conversion Rad to Deg/1

== system schemat_koncowy_irp/Position 4/Filters 4 ==
  Sin && Cos : Inport
  Analog Butterworth LP Filter : Subsystem  mask(buttap){Parameter3=2*pi*16, Parameter4=1}
      mask prompts: Parameter3 "Cutoff frequency (rad/sec)"; Parameter4 "Order"
      mask help:
      | Analog Butterworth low pass filter.
      |
      | (Requires Signal Processing Toolbox)
      mask init:
      | [z,p,k]=buttap(@2); z=@1*z; p=@1*p; k=real(prod(-p)); [num,den]=zp2tf(z,p,k); w=logspace(log10(@1/10),log10(10*@1),20); h=freqs(num,den,w);
      mask Help: Butterworth low pass filter using MATLAB's butter command.
      mask Display: plot(20*log10(w),20*log10(abs(h)))
  Analog Butterworth LP Filter1 : Subsystem  mask(buttap){Parameter3=2*pi*16, Parameter4=1}
      mask prompts: Parameter3 "Cutoff frequency (rad/sec)"; Parameter4 "Order"
      mask help:
      | Analog Butterworth low pass filter.
      |
      | (Requires Signal Processing Toolbox)
      mask init:
      | [z,p,k]=buttap(@2); z=@1*z; p=@1*p; k=real(prod(-p)); [num,den]=zp2tf(z,p,k); w=logspace(log10(@1/10),log10(10*@1),20); h=freqs(num,den,w);
      mask Help: Butterworth low pass filter using MATLAB's butter command.
      mask Display: plot(20*log10(w),20*log10(abs(h)))
  Demux : Demux  Outputs=2
  Sin : Outport
  Cos : Outport  Port=2
  wires:
  Analog Butterworth LP Filter/1(Out1) -> Sin/1
  Analog Butterworth LP Filter1/1(Out1) -> Cos/1
  Sin && Cos/1 -> Demux/1
  Demux/1 -> Analog Butterworth LP Filter/1(In1)
  Demux/2 -> Analog Butterworth LP Filter1/1(In1)

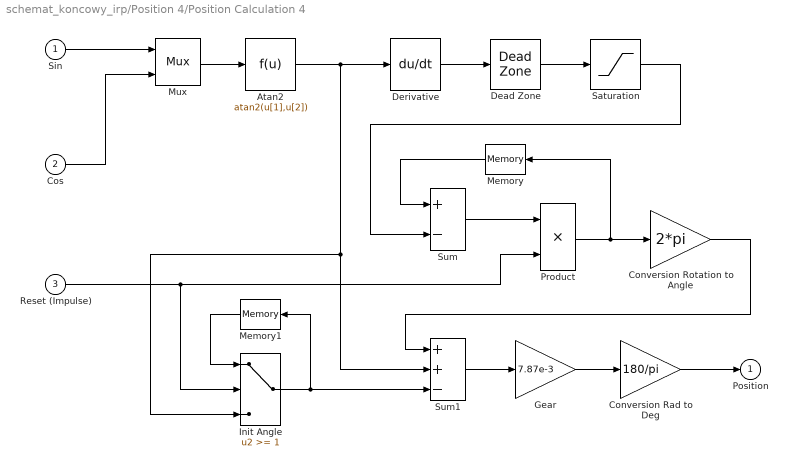
== system schemat_koncowy_irp/Position 4/Position Calculation 4 ==
  Sin : Inport
  Cos : Inport  Port=2
  Reset (Impulse) : Inport  Port=3
  Atan2 : Fcn  Expr=atan2(u[1],u[2])
  Conversion Rad to Deg : Gain  Gain=180/pi  SaturateOnIntegerOverflow=on  OutDataTypeStr=Inherit: Same as input  ParamDataTypeStr=Inherit: Same as input
  Conversion Rotation to Angle : Gain  Gain=2*pi  SaturateOnIntegerOverflow=on  OutDataTypeStr=Inherit: Same as input  ParamDataTypeStr=Inherit: Same as input
  Dead Zone : DeadZone  LowerValue=-5000  UpperValue=5000  SaturateOnIntegerOverflow=on
  Derivative : Derivative
  Gear : Gain  Gain=7.87e-3  SaturateOnIntegerOverflow=on  OutDataTypeStr=Inherit: Same as input  ParamDataTypeStr=Inherit: Same as input
  Init Angle : Switch  Threshold=1  SaturateOnIntegerOverflow=on  InputSameDT=on
  Memory : Memory
  Memory1 : Memory
  Mux : Mux  Inputs=2
  Product : Product  SaturateOnIntegerOverflow=on  RndMeth=Zero  InputSameDT=on  OutDataTypeStr=Inherit: Same as first input
  Saturation : Saturate  UpperLimit=1  LowerLimit=-1
  Sum : Sum  Inputs=+-  SaturateOnIntegerOverflow=on  InputSameDT=on  OutDataTypeStr=Inherit: Same as first input
  Sum1 : Sum  Inputs=++-  SaturateOnIntegerOverflow=on  InputSameDT=on  OutDataTypeStr=Inherit: Same as first input
  Position : Outport
  wires:
  Gear/1 -> Conversion Rad to Deg/1
  Sum1/1 -> Gear/1
  Sum/1 -> Product/1
  Dead Zone/1 -> Saturation/1
  Derivative/1 -> Dead Zone/1
  Mux/1 -> Atan2/1
  Sin/1 -> Mux/1
  Conversion Rad to Deg/1 -> Position/1
  Saturation/1 -> Sum/2
  Conversion Rotation to Angle/1 -> Sum1/1
  Reset (Impulse)/1 -> Product/2, Init Angle/2
  Atan2/1 -> Derivative/1, Sum1/2, Init Angle/3
  Cos/1 -> Mux/2
  Memory/1 -> Sum/1
  Product/1 -> Conversion Rotation to Angle/1, Memory/1
  Memory1/1 -> Init Angle/1
  Init Angle/1 -> Sum1/3, Memory1/1

== system schemat_koncowy_irp/Position 5/Filters 5 ==
  Sin && Cos : Inport
  Analog Butterworth LP Filter : Subsystem  mask(buttap){Parameter3=2*pi*16, Parameter4=1}
      mask prompts: Parameter3 "Cutoff frequency (rad/sec)"; Parameter4 "Order"
      mask help:
      | Analog Butterworth low pass filter.
      |
      | (Requires Signal Processing Toolbox)
      mask init:
      | [z,p,k]=buttap(@2); z=@1*z; p=@1*p; k=real(prod(-p)); [num,den]=zp2tf(z,p,k); w=logspace(log10(@1/10),log10(10*@1),20); h=freqs(num,den,w);
      mask Help: Butterworth low pass filter using MATLAB's butter command.
      mask Display: plot(20*log10(w),20*log10(abs(h)))
  Analog Butterworth LP Filter1 : Subsystem  mask(buttap){Parameter3=2*pi*16, Parameter4=1}
      mask prompts: Parameter3 "Cutoff frequency (rad/sec)"; Parameter4 "Order"
      mask help:
      | Analog Butterworth low pass filter.
      |
      | (Requires Signal Processing Toolbox)
      mask init:
      | [z,p,k]=buttap(@2); z=@1*z; p=@1*p; k=real(prod(-p)); [num,den]=zp2tf(z,p,k); w=logspace(log10(@1/10),log10(10*@1),20); h=freqs(num,den,w);
      mask Help: Butterworth low pass filter using MATLAB's butter command.
      mask Display: plot(20*log10(w),20*log10(abs(h)))
  Demux : Demux  Outputs=2
  Sin : Outport
  Cos : Outport  Port=2
  wires:
  Analog Butterworth LP Filter/1(Out1) -> Sin/1
  Analog Butterworth LP Filter1/1(Out1) -> Cos/1
  Sin && Cos/1 -> Demux/1
  Demux/1 -> Analog Butterworth LP Filter/1(In1)
  Demux/2 -> Analog Butterworth LP Filter1/1(In1)

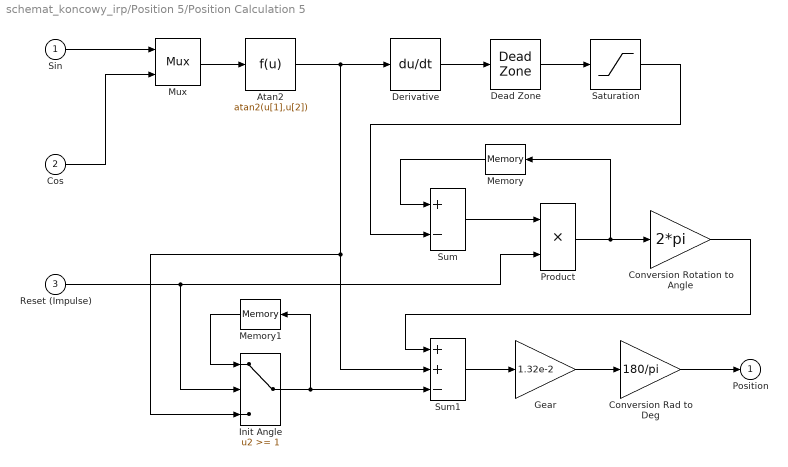
== system schemat_koncowy_irp/Position 5/Position Calculation 5 ==
  Sin : Inport
  Cos : Inport  Port=2
  Reset (Impulse) : Inport  Port=3
  Atan2 : Fcn  Expr=atan2(u[1],u[2])
  Conversion Rad to Deg : Gain  Gain=180/pi  SaturateOnIntegerOverflow=on  OutDataTypeStr=Inherit: Same as input  ParamDataTypeStr=Inherit: Same as input
  Conversion Rotation to Angle : Gain  Gain=2*pi  SaturateOnIntegerOverflow=on  OutDataTypeStr=Inherit: Same as input  ParamDataTypeStr=Inherit: Same as input
  Dead Zone : DeadZone  LowerValue=-5000  UpperValue=5000  SaturateOnIntegerOverflow=on
  Derivative : Derivative
  Gear : Gain  Gain=1.32e-2  SaturateOnIntegerOverflow=on  OutDataTypeStr=Inherit: Same as input  ParamDataTypeStr=Inherit: Same as input
  Init Angle : Switch  Threshold=1  SaturateOnIntegerOverflow=on  InputSameDT=on
  Memory : Memory
  Memory1 : Memory
  Mux : Mux  Inputs=2
  Product : Product  SaturateOnIntegerOverflow=on  RndMeth=Zero  InputSameDT=on  OutDataTypeStr=Inherit: Same as first input
  Saturation : Saturate  UpperLimit=1  LowerLimit=-1
  Sum : Sum  Inputs=+-  SaturateOnIntegerOverflow=on  InputSameDT=on  OutDataTypeStr=Inherit: Same as first input
  Sum1 : Sum  Inputs=++-  SaturateOnIntegerOverflow=on  InputSameDT=on  OutDataTypeStr=Inherit: Same as first input
  Position : Outport
  wires:
  Gear/1 -> Conversion Rad to Deg/1
  Sum1/1 -> Gear/1
  Sum/1 -> Product/1
  Dead Zone/1 -> Saturation/1
  Derivative/1 -> Dead Zone/1
  Mux/1 -> Atan2/1
  Sin/1 -> Mux/1
  Conversion Rad to Deg/1 -> Position/1
  Saturation/1 -> Sum/2
  Conversion Rotation to Angle/1 -> Sum1/1
  Reset (Impulse)/1 -> Product/2, Init Angle/2
  Atan2/1 -> Derivative/1, Sum1/2, Init Angle/3
  Cos/1 -> Mux/2
  Memory/1 -> Sum/1
  Product/1 -> Conversion Rotation to Angle/1, Memory/1
  Memory1/1 -> Init Angle/1
  Init Angle/1 -> Sum1/3, Memory1/1

== system schemat_koncowy_irp/RTI Data/RTI Data Store ==
  RTI Data Store : Subsystem  mask(RTI_DATA_STORE){}
      mask help:
      | RTI Data Store Block. This block is used by RTI to store internal model dependent data. Deleting this block will result in data loss.
      |
      | NEVER DELETE, COPY, OR MODIFY THIS BLOCK!
      mask Help:
      | RTI Data Store Block. This block is used by RTI to store internal model dependent data. Deleting this block will result in data loss.
      | 
      | NEVER DELETE, COPY, OR MODIFY THIS BLOCK!
      mask Display: text(0.5, 0.5, ' ', 'HorizontalAlignment', 'center');

== system schemat_koncowy_irp/Position 1/Filters 1/Analog Butterworth LP Filter ==
  In1 : Inport
  Analog Butterworth LP Filter : ZeroPole  Zeros=z  Poles=p  Gain=k
  Out1 : Outport
  wires:
  Analog Butterworth LP Filter/1 -> Out1/1
  In1/1 -> Analog Butterworth LP Filter/1
